simulink model "Charts"  (R2013a)
settings: Solver=ode45  StartTime=0.0  StopTime=5  RelTol=1e-3
undefined symbols (not defined in the file or in its folder): sigbuilder_block
settings Model: Creator=Daniel  LastModifiedBy=Daniel

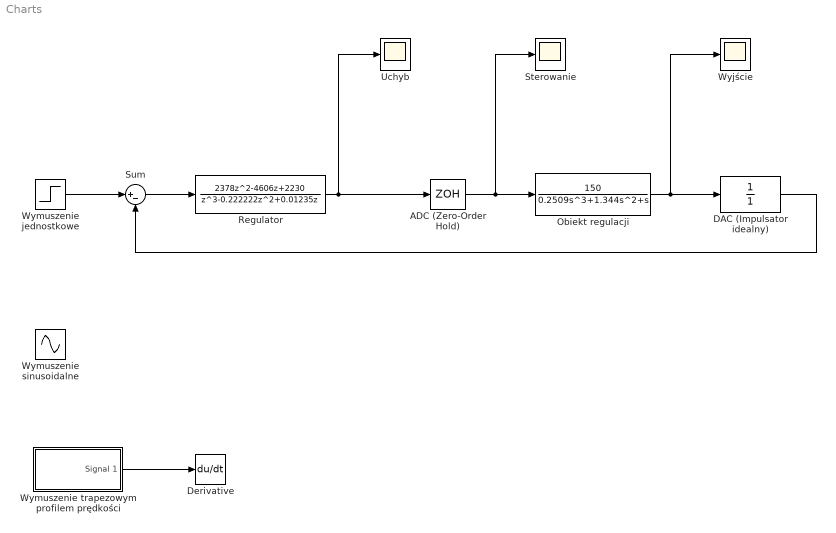
== system Charts ==
  ADC (Zero-Order Hold) : ZeroOrderHold
  DAC (Impulsator idealny) : DiscreteTransferFcn  Denominator=[1]  SampleTime=0.004
  Derivative : Derivative
  Obiekt regulacji : TransferFcn  Numerator=[150]  Denominator=[0.2509 1.344 1 0]
  Regulator : DiscreteTransferFcn  Numerator=[2378 -4606 +2230]  Denominator=[1 -0.222222 0.01235 0]  SampleTime=0.004
  Sterowanie : Scope
  Sum : Sum  Inputs=|+-
  Uchyb : Scope
      settings: SaveName=ScopeData2
  Wyjście : Scope
  Wymuszenie jednostkowe : Step  SampleTime=0
  Wymuszenie sinusoidalne : Sin  SampleTime=0
  Wymuszenie trapezowym profilem prędkości : Subsystem  Tag=STV Subsys  LoadFcn=sigbuilder_block('load');  StartFcn=sigbuilder_block('start');  StopFcn=sigbuilder_block('stop');  ClipboardFcn=sigbuilder_block('clipboard');  mask(Sigbuilder block){}
      mask help: Simulink:masks:SigbuilderBlock_MD
      mask init:
      | if ~strcmp(get_param(bdroot(gcbh),'SimulationStatus'),'stopped') tuvar = sigbuilder_block('maskInit'); end
      settings: CopyFcn=sigbuilder_block('copy');  DeleteFcn=sigbuilder_block('delete');  ModelCloseFcn=sigbuilder_block('modelClose');  PreSaveFcn=sigbuilder_block('preSave');  PauseFcn=sigbuilder_block('pause');  ContinueFcn=sigbuilder_block('continue');  NameChangeFcn=sigbuilder_block('namechange');  OpenFcn=sigbuilder_block('open',[104.25 131.25 550.5 399.75 ]);  CloseFcn=sigbuilder_block('close');
      mask Display: plot(0, 0, 100, 100,[2, 2, 32, 32, 2], [68, 8, 8, 68, 68],[32, 2], [38, 38], [32, 19, 2],[53, 60, 44], [32, 17, 17, 2],[16, 16, 31, 31]);txt = getActiveGroup(gcbh);text(2, 100, txt,'verticalAlignment', 'top');
  wires:
  ADC (Zero-Order Hold)/1 -> Obiekt regulacji/1, Sterowanie/1
  Obiekt regulacji/1 -> Wyjście/1, DAC (Impulsator idealny)/1
  Regulator/1 -> Uchyb/1, ADC (Zero-Order Hold)/1
  Sum/1 -> Regulator/1
  DAC (Impulsator idealny)/1 -> Sum/2
  Wymuszenie jednostkowe/1 -> Sum/1
  Wymuszenie trapezowym profilem prędkości/1(Signal 1) -> Derivative/1

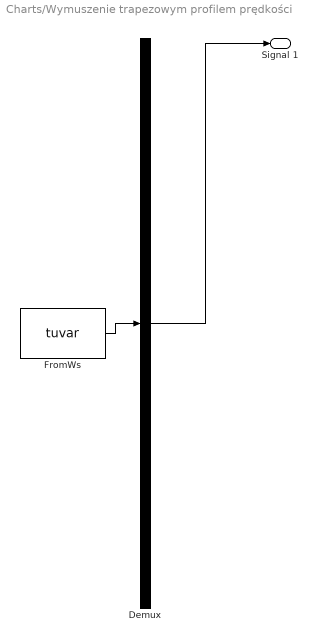
== system Charts/Wymuszenie trapezowym profilem prędkości ==
  Demux : Demux  Tag=STV Demux  Outputs=1
  FromWs : FromWorkspace  Tag=STV FromWs  VariableName=tuvar  SampleTime=0
      SigBuilderData=|
      | common.afterFinalStr = 'Extrapolate'
      | common.sampleTime = 0
      | dataSet.timeRange = [0 10]
      | dataSet.name = 'Group 1'
      | sbobj.Groups.Name = 'Group 1'
      | sbobj.Groups.Signals.Name = 'Signal 1'
      | sbobj.Groups.Signals.XData = [0 4 6 6 10]
      | sbobj.Groups.Signals.YData = [0 0.995 1 0.995 0]
  Signal 1 : Outport  Tag=STV Outport
  wires:
  Demux/1 -> Signal 1/1
  FromWs/1 -> Demux/1
